simulink model "RBF_NN_controller"  (R2021b)
settings: Solver=ode45  StartTime=0.0  StopTime=40  FixedStep=0.1  RelTol=1e-5  EnableMultiTasking=on
settings Model: Creator=Admin  LastModifiedBy=Admin
settings DataIOCC: SaveFormat=Array  SignalLoggingSaveFormat=ModelDataLogs  ReturnWorkspaceOutputs=off  SignalLoggingName=sigsOut
settings OptimizationCC: BooleanDataType=off
settings DebuggingCC: SaveWithParameterizedLinksMsg=none  UnderspecifiedInitializationDetection=Classic  MergeDetectMultiDrivingBlocksExec=none  SignalResolutionControl=TryResolveAllWithWarning  MultiTaskDSMMsg=warning  MultiTaskCondExecSysMsg=none
settings HardwareCC: ProdBitPerPointer=32  ProdBitPerSizeT=32  ProdBitPerPtrDiffT=32  ProdLargestAtomicFloat=None  ProdIntDivRoundTo=Undefined  ProdEndianess=Unspecified  ProdWordSize=32  ProdHWDeviceType=32-bit Generic  TargetUnknown=on
settings ModelReferenceCC: PropagateSignalLabelsOutOfModel=off
settings GRTTargetCC: CombineOutputUpdateFcns=off  GRTInterface=on
settings ConfigComp: CovMetricSettings=dw  CovSaveCumulativeToWorkspaceVar=on  CovSaveSingleToWorkspaceVar=on

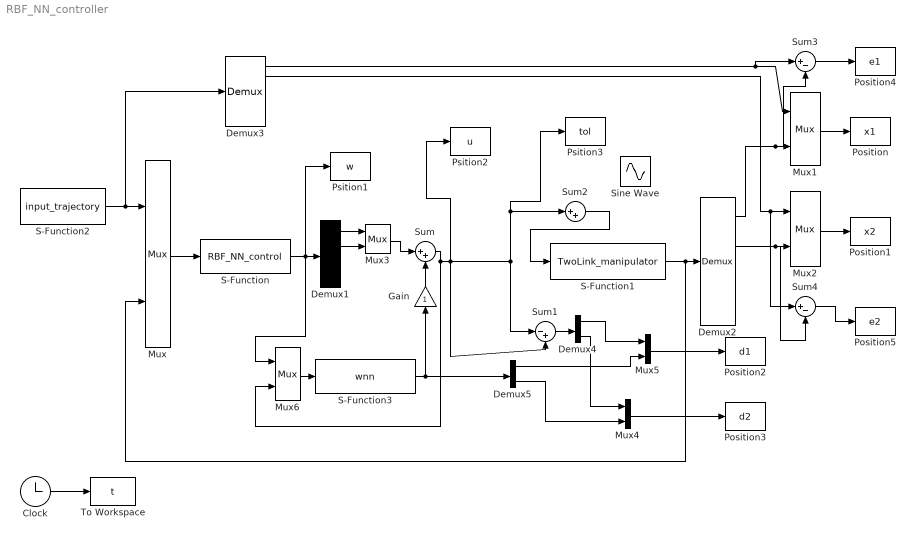
== system RBF_NN_controller ==
  Clock : Clock
  Demux1 : Demux
      settings: DisplayOption=none
  Demux2 : Demux
      settings: DisplayOption=none
  Demux3 : Demux  Outputs=6
      settings: DisplayOption=none
  Demux4 : Demux  Outputs=2
  Demux5 : Demux  Outputs=2
  Gain : Gain  SaturateOnIntegerOverflow=on  OutDataTypeStr=Inherit: Same as input  ParamDataTypeStr=Inherit: Same as input
  Mux{,1..6} (7 alike) : Mux  Inputs=2
  Position : ToWorkspace  VariableName=x1  SampleTime=-1
  Position1 : ToWorkspace  VariableName=x2  SampleTime=-1
  Position2 : ToWorkspace  VariableName=d1  SampleTime=-1
  Position3 : ToWorkspace  VariableName=d2  SampleTime=-1
  Position4 : ToWorkspace  VariableName=e1  SampleTime=-1
  Position5 : ToWorkspace  VariableName=e2  SampleTime=-1
  Psition1 : ToWorkspace  VariableName=w  SampleTime=-1
  Psition2 : ToWorkspace  VariableName=u  SampleTime=-1
  Psition3 : ToWorkspace  VariableName=tol  SampleTime=-1
  S-Function : S-Function  FunctionName=RBF_NN_control  SFunctionDeploymentMode=off  EnableBusSupport=off
  S-Function1 : S-Function  FunctionName=TwoLink_manipulator  SFunctionDeploymentMode=off  EnableBusSupport=off
  S-Function2 : S-Function  FunctionName=input_trajectory  SFunctionDeploymentMode=off  EnableBusSupport=off
  S-Function3 : S-Function  FunctionName=wnn  SFunctionDeploymentMode=off  EnableBusSupport=off
  Sine Wave : Sin  Amplitude=[20;20]  Bias=[0;0]  Frequency=[0.5;0.5]  Phase=[5;5]  SampleTime=0
  Sum : Sum  Inputs=|++  SaturateOnIntegerOverflow=on
  Sum1 : Sum  Inputs=|-+  SaturateOnIntegerOverflow=on
  Sum2 : Sum  Inputs=|++  SaturateOnIntegerOverflow=on
  Sum3 : Sum  Inputs=|+-
  Sum4 : Sum  Inputs=|+-
  To Workspace : ToWorkspace  VariableName=t  SampleTime=-1
  wires:
  S-Function/1 -> Demux1/1, Psition1/1, Mux6/1
  Demux2/1 -> Sum3/2, Mux1/2
  S-Function2/1 -> Demux3/1, Mux/1
  Demux2/2 -> Sum4/2, Mux2/2
  Demux3/1 -> Sum3/1, Mux1/1
  Demux3/2 -> Sum4/1, Mux2/1
  S-Function1/1 -> Mux/2, Demux2/1
  Demux1/1 -> Mux3/1
  Demux1/2 -> Mux3/2
  Sum/1 -> Sum2/1, Psition3/1, Sum1/1, Sum1/2, Psition2/1, Mux6/2
  Mux3/1 -> Sum/1
  S-Function3/1 -> Gain/1, Demux5/1
  Mux6/1 -> S-Function3/1
  Mux1/1 -> Position/1
  Mux2/1 -> Position1/1
  Mux/1 -> S-Function/1
  Mux5/1 -> Position2/1
  Gain/1 -> Sum/2
  Sum1/1 -> Demux4/1
  Demux4/1 -> Mux5/1
  Demux5/1 -> Mux5/2
  Mux4/1 -> Position3/1
  Demux4/2 -> Mux4/1
  Demux5/2 -> Mux4/2
  Clock/1 -> To Workspace/1
  Sum2/1 -> S-Function1/1
  Sum3/1 -> Position4/1
  Sum4/1 -> Position5/1
